simulink model "PIDRegulaceSS"  (R2020b)
settings: Solver=VariableStepAuto  StartTime=0.0  StopTime=inf  RelTol=1e-3
undefined symbols (not defined in the file): A_num, B_num, C, D, g, L
libraries: pid_lib x8, simulink x4
settings Model: Creator=kpass  LastModifiedBy=kpass

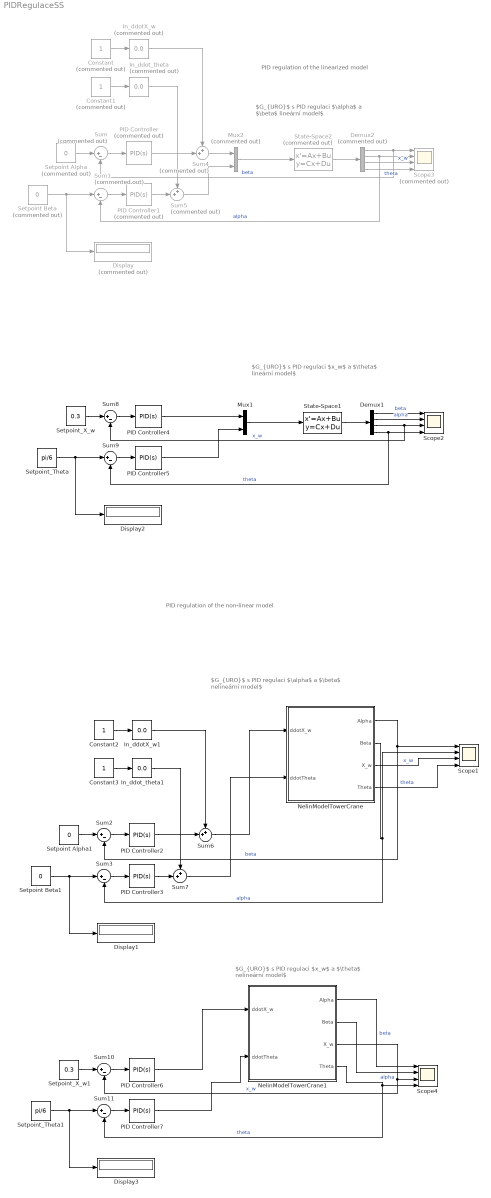
== system PIDRegulaceSS ==
  note: $G_{URO}$ s PID regulaci $x_w$ a $\theta$ nelineární model$
  note: PID regulation of the linearized model
  note: PID regulation of the non-linear model
  note: $G_{URO}$ s PID regulaci $x_w$ a $\theta$ lineární model$
  note: $G_{URO}$ s PID regulaci $\alpha$ a $\beta$ nelineární model$
  note: $G_{URO}$ s PID regulaci $\alpha$ a $\beta$ lineární model$
  Constant : Constant  Commented=on
  Constant1 : Constant  Commented=on
  Constant2 : Constant
  Constant3 : Constant
  Demux1 : Demux
  Demux2 : Demux  Commented=on
  Display : Display  Commented=on
  Display1 : Display
  Display2 : Display
  Display3 : Display
  In_ddotX_w : simulink/Math Operations/Slider Gain  Commented=on  gain=0.0  low=0  high=0.1
  In_ddotX_w1 : simulink/Math Operations/Slider Gain  gain=0.0  low=0  high=0.1
  In_ddot_theta : simulink/Math Operations/Slider Gain  Commented=on  gain=0.0  low=0  high=0.1
  In_ddot_theta1 : simulink/Math Operations/Slider Gain  gain=0.0  low=0  high=0.1
  Mux1 : Mux  Inputs=2
  Mux2 : Mux  Commented=on  Inputs=2
  NelinModelTowerCrane : Subsystem
  NelinModelTowerCrane1 : Subsystem
  PID Controller : pid_lib/PID Controller  Commented=on  Controller=PID  Form=Parallel  TimeDomain=Continuous-time  UseExternalTs=off  SampleTime=-1  IntegratorMethod=Forward Euler  FilterMethod=Forward Euler  ControllerParametersSource=internal  P=1  I=0  D=0  UseFilter=on  N=100  TunerSelectOption=Transfer Function Based (PID Tuner App)  InitialConditionSource=internal  InitialConditionForIntegrator=0  InitialConditionForFilter=0  DifferentiatorICPrevScaledInput=0  ExternalReset=none  TrackingMode=off  Kt=1  LimitOutput=off  SatLimitsSource=internal  UpperSaturationLimit=inf  LowerSaturationLimit=-inf  LinearizeAsGain=on  AntiWindupMode=none  Kb=1  POutMin=[]  POutMax=[]  IOutMin=[]  IOutMax=[]  DOutMin=[]  DOutMax=[]  NOutMin=[]  NOutMax=[]  SumOutMin=[]  SumOutMax=[]  SaturationOutMin=[]  SaturationOutMax=[]  PParamMin=[]  PParamMax=[]  IParamMin=[]  IParamMax=[]  DParamMin=[]  DParamMax=[]  NParamMin=[]  NParamMax=[]  KbParamMin=[]  KbParamMax=[]  KtParamMin=[]  KtParamMax=[]  KbOutMin=[]  KbOutMax=[]  KtOutMin=[]  KtOutMax=[]  IntegratorOutMin=[]  IntegratorOutMax=[]  FilterOutMin=[]  FilterOutMax=[]  SumI1OutMin=[]  SumI1OutMax=[]  SumI2OutMin=[]  SumI2OutMax=[]  SumI3OutMin=[]  SumI3OutMax=[]  SumI4OutMin=[]  SumI4OutMax=[]  SumDOutMin=[]  SumDOutMax=[]  DifferentiatorOutMin=[]  DifferentiatorOutMax=[]  FilterDiffOutCoefMin=[]  FilterDiffOutCoefMax=[]  ReciprocalOutMin=[]  ReciprocalOutMax=[]  SumDenOutMin=[]  SumDenOutMax=[]  SumNumOutMin=[]  SumNumOutMax=[]  DivideOutMin=[]  DivideOutMax=[]  UdiffTsProdOutMin=[]  UdiffTsProdOutMax=[]  NTsProdOutMin=[]  NTsProdOutMax=[]  UintegralTsProdOutMin=[]  UintegralTsProdOutMax=[]  UngainTsProdOutMin=[]  UngainTsProdOutMax=[]  IntegratorContinuousStateAttributes=''  IntegratorStateMustResolveToSignalObject=off  IntegratorRTWStateStorageClass=Auto  FilterContinuousStateAttributes=''  FilterStateMustResolveToSignalObject=off  FilterRTWStateStorageClass=Auto  ParallelPVariant=InternalParameters  IdealPVariant=Disabled  IVariant=InternalParameters  DVariant=InternalParameters  IntegratorVariant=Continuous  SatVariant=Disabled  AWVariant=Passthrough  PCopyVariant=Disabled  TRVariant=Disabled  FdbkBlocksVariant=Forward  IdealPFdbkVariant=Disabled  SatFdbkVariant=Disabled  DerivativeFilterVariant=ContFilter  NVariant=InternalParameters  NCopyVariant=Disabled  FilterICVariant=InternalICsFilter  IntegratorICVariant=InternalICs  ExternalResetVariant=Disabled  TRSumVariant=Passthrough  SumFdbkVariant=Disabled  SumVariant=Sum_PID  TsampFilterVariant=InternalTs  TsampNgainVariant=Passthrough  TsampIntegralVariant=Passthrough  ExternalSaturationOutDataTypeStr=Inherit: Same as second input
  PID Controller1 : pid_lib/PID Controller  Commented=on  Controller=PID  Form=Parallel  TimeDomain=Continuous-time  UseExternalTs=off  SampleTime=-1  IntegratorMethod=Forward Euler  FilterMethod=Forward Euler  ControllerParametersSource=internal  P=1  I=0  D=0  UseFilter=on  N=100  TunerSelectOption=Transfer Function Based (PID Tuner App)  InitialConditionSource=internal  InitialConditionForIntegrator=0  InitialConditionForFilter=0  DifferentiatorICPrevScaledInput=0  ExternalReset=none  TrackingMode=off  Kt=1  LimitOutput=off  SatLimitsSource=internal  UpperSaturationLimit=inf  LowerSaturationLimit=-inf  LinearizeAsGain=on  AntiWindupMode=none  Kb=1  POutMin=[]  POutMax=[]  IOutMin=[]  IOutMax=[]  DOutMin=[]  DOutMax=[]  NOutMin=[]  NOutMax=[]  SumOutMin=[]  SumOutMax=[]  SaturationOutMin=[]  SaturationOutMax=[]  PParamMin=[]  PParamMax=[]  IParamMin=[]  IParamMax=[]  DParamMin=[]  DParamMax=[]  NParamMin=[]  NParamMax=[]  KbParamMin=[]  KbParamMax=[]  KtParamMin=[]  KtParamMax=[]  KbOutMin=[]  KbOutMax=[]  KtOutMin=[]  KtOutMax=[]  IntegratorOutMin=[]  IntegratorOutMax=[]  FilterOutMin=[]  FilterOutMax=[]  SumI1OutMin=[]  SumI1OutMax=[]  SumI2OutMin=[]  SumI2OutMax=[]  SumI3OutMin=[]  SumI3OutMax=[]  SumI4OutMin=[]  SumI4OutMax=[]  SumDOutMin=[]  SumDOutMax=[]  DifferentiatorOutMin=[]  DifferentiatorOutMax=[]  FilterDiffOutCoefMin=[]  FilterDiffOutCoefMax=[]  ReciprocalOutMin=[]  ReciprocalOutMax=[]  SumDenOutMin=[]  SumDenOutMax=[]  SumNumOutMin=[]  SumNumOutMax=[]  DivideOutMin=[]  DivideOutMax=[]  UdiffTsProdOutMin=[]  UdiffTsProdOutMax=[]  NTsProdOutMin=[]  NTsProdOutMax=[]  UintegralTsProdOutMin=[]  UintegralTsProdOutMax=[]  UngainTsProdOutMin=[]  UngainTsProdOutMax=[]  IntegratorContinuousStateAttributes=''  IntegratorStateMustResolveToSignalObject=off  IntegratorRTWStateStorageClass=Auto  FilterContinuousStateAttributes=''  FilterStateMustResolveToSignalObject=off  FilterRTWStateStorageClass=Auto  ParallelPVariant=InternalParameters  IdealPVariant=Disabled  IVariant=InternalParameters  DVariant=InternalParameters  IntegratorVariant=Continuous  SatVariant=Disabled  AWVariant=Passthrough  PCopyVariant=Disabled  TRVariant=Disabled  FdbkBlocksVariant=Forward  IdealPFdbkVariant=Disabled  SatFdbkVariant=Disabled  DerivativeFilterVariant=ContFilter  NVariant=InternalParameters  NCopyVariant=Disabled  FilterICVariant=InternalICsFilter  IntegratorICVariant=InternalICs  ExternalResetVariant=Disabled  TRSumVariant=Passthrough  SumFdbkVariant=Disabled  SumVariant=Sum_PID  TsampFilterVariant=InternalTs  TsampNgainVariant=Passthrough  TsampIntegralVariant=Passthrough  ExternalSaturationOutDataTypeStr=Inherit: Same as second input
  PID Controller2 : pid_lib/PID Controller  Controller=PID  Form=Parallel  TimeDomain=Continuous-time  UseExternalTs=off  SampleTime=-1  IntegratorMethod=Forward Euler  FilterMethod=Forward Euler  ControllerParametersSource=internal  P=1  I=0  D=49.05  UseFilter=on  N=10  TunerSelectOption=Transfer Function Based (PID Tuner App)  InitialConditionSource=internal  InitialConditionForIntegrator=0  InitialConditionForFilter=0  DifferentiatorICPrevScaledInput=0  ExternalReset=none  TrackingMode=off  Kt=1  LimitOutput=off  SatLimitsSource=internal  UpperSaturationLimit=inf  LowerSaturationLimit=-inf  LinearizeAsGain=on  AntiWindupMode=none  Kb=1  POutMin=[]  POutMax=[]  IOutMin=[]  IOutMax=[]  DOutMin=[]  DOutMax=[]  NOutMin=[]  NOutMax=[]  SumOutMin=[]  SumOutMax=[]  SaturationOutMin=[]  SaturationOutMax=[]  PParamMin=[]  PParamMax=[]  IParamMin=[]  IParamMax=[]  DParamMin=[]  DParamMax=[]  NParamMin=[]  NParamMax=[]  KbParamMin=[]  KbParamMax=[]  KtParamMin=[]  KtParamMax=[]  KbOutMin=[]  KbOutMax=[]  KtOutMin=[]  KtOutMax=[]  IntegratorOutMin=[]  IntegratorOutMax=[]  FilterOutMin=[]  FilterOutMax=[]  SumI1OutMin=[]  SumI1OutMax=[]  SumI2OutMin=[]  SumI2OutMax=[]  SumI3OutMin=[]  SumI3OutMax=[]  SumI4OutMin=[]  SumI4OutMax=[]  SumDOutMin=[]  SumDOutMax=[]  DifferentiatorOutMin=[]  DifferentiatorOutMax=[]  FilterDiffOutCoefMin=[]  FilterDiffOutCoefMax=[]  ReciprocalOutMin=[]  ReciprocalOutMax=[]  SumDenOutMin=[]  SumDenOutMax=[]  SumNumOutMin=[]  SumNumOutMax=[]  DivideOutMin=[]  DivideOutMax=[]  UdiffTsProdOutMin=[]  UdiffTsProdOutMax=[]  NTsProdOutMin=[]  NTsProdOutMax=[]  UintegralTsProdOutMin=[]  UintegralTsProdOutMax=[]  UngainTsProdOutMin=[]  UngainTsProdOutMax=[]  IntegratorContinuousStateAttributes=''  IntegratorStateMustResolveToSignalObject=off  IntegratorRTWStateStorageClass=Auto  FilterContinuousStateAttributes=''  FilterStateMustResolveToSignalObject=off  FilterRTWStateStorageClass=Auto  ParallelPVariant=InternalParameters  IdealPVariant=Disabled  IVariant=InternalParameters  DVariant=InternalParameters  IntegratorVariant=Continuous  SatVariant=Disabled  AWVariant=Passthrough  PCopyVariant=Disabled  TRVariant=Disabled  FdbkBlocksVariant=Forward  IdealPFdbkVariant=Disabled  SatFdbkVariant=Disabled  DerivativeFilterVariant=ContFilter  NVariant=InternalParameters  NCopyVariant=Disabled  FilterICVariant=InternalICsFilter  IntegratorICVariant=InternalICs  ExternalResetVariant=Disabled  TRSumVariant=Passthrough  SumFdbkVariant=Disabled  SumVariant=Sum_PID  TsampFilterVariant=InternalTs  TsampNgainVariant=Passthrough  TsampIntegralVariant=Passthrough  ExternalSaturationOutDataTypeStr=Inherit: Same as second input
  PID Controller3 : pid_lib/PID Controller  Controller=PID  Form=Parallel  TimeDomain=Continuous-time  UseExternalTs=off  SampleTime=-1  IntegratorMethod=Forward Euler  FilterMethod=Forward Euler  ControllerParametersSource=internal  P=1  I=0  D=49.05  UseFilter=on  N=10  TunerSelectOption=Transfer Function Based (PID Tuner App)  InitialConditionSource=internal  InitialConditionForIntegrator=0  InitialConditionForFilter=0  DifferentiatorICPrevScaledInput=0  ExternalReset=none  TrackingMode=off  Kt=1  LimitOutput=off  SatLimitsSource=internal  UpperSaturationLimit=inf  LowerSaturationLimit=-inf  LinearizeAsGain=on  AntiWindupMode=none  Kb=1  POutMin=[]  POutMax=[]  IOutMin=[]  IOutMax=[]  DOutMin=[]  DOutMax=[]  NOutMin=[]  NOutMax=[]  SumOutMin=[]  SumOutMax=[]  SaturationOutMin=[]  SaturationOutMax=[]  PParamMin=[]  PParamMax=[]  IParamMin=[]  IParamMax=[]  DParamMin=[]  DParamMax=[]  NParamMin=[]  NParamMax=[]  KbParamMin=[]  KbParamMax=[]  KtParamMin=[]  KtParamMax=[]  KbOutMin=[]  KbOutMax=[]  KtOutMin=[]  KtOutMax=[]  IntegratorOutMin=[]  IntegratorOutMax=[]  FilterOutMin=[]  FilterOutMax=[]  SumI1OutMin=[]  SumI1OutMax=[]  SumI2OutMin=[]  SumI2OutMax=[]  SumI3OutMin=[]  SumI3OutMax=[]  SumI4OutMin=[]  SumI4OutMax=[]  SumDOutMin=[]  SumDOutMax=[]  DifferentiatorOutMin=[]  DifferentiatorOutMax=[]  FilterDiffOutCoefMin=[]  FilterDiffOutCoefMax=[]  ReciprocalOutMin=[]  ReciprocalOutMax=[]  SumDenOutMin=[]  SumDenOutMax=[]  SumNumOutMin=[]  SumNumOutMax=[]  DivideOutMin=[]  DivideOutMax=[]  UdiffTsProdOutMin=[]  UdiffTsProdOutMax=[]  NTsProdOutMin=[]  NTsProdOutMax=[]  UintegralTsProdOutMin=[]  UintegralTsProdOutMax=[]  UngainTsProdOutMin=[]  UngainTsProdOutMax=[]  IntegratorContinuousStateAttributes=''  IntegratorStateMustResolveToSignalObject=off  IntegratorRTWStateStorageClass=Auto  FilterContinuousStateAttributes=''  FilterStateMustResolveToSignalObject=off  FilterRTWStateStorageClass=Auto  ParallelPVariant=InternalParameters  IdealPVariant=Disabled  IVariant=InternalParameters  DVariant=InternalParameters  IntegratorVariant=Continuous  SatVariant=Disabled  AWVariant=Passthrough  PCopyVariant=Disabled  TRVariant=Disabled  FdbkBlocksVariant=Forward  IdealPFdbkVariant=Disabled  SatFdbkVariant=Disabled  DerivativeFilterVariant=ContFilter  NVariant=InternalParameters  NCopyVariant=Disabled  FilterICVariant=InternalICsFilter  IntegratorICVariant=InternalICs  ExternalResetVariant=Disabled  TRSumVariant=Passthrough  SumFdbkVariant=Disabled  SumVariant=Sum_PID  TsampFilterVariant=InternalTs  TsampNgainVariant=Passthrough  TsampIntegralVariant=Passthrough  ExternalSaturationOutDataTypeStr=Inherit: Same as second input
  PID Controller{4..7} (4 alike) : pid_lib/PID Controller  Controller=PID  Form=Parallel  TimeDomain=Continuous-time  UseExternalTs=off  SampleTime=-1  IntegratorMethod=Forward Euler  FilterMethod=Forward Euler  ControllerParametersSource=internal  P=1  I=0  D=2  UseFilter=on  N=100  TunerSelectOption=Transfer Function Based (PID Tuner App)  InitialConditionSource=internal  InitialConditionForIntegrator=0  InitialConditionForFilter=0  DifferentiatorICPrevScaledInput=0  ExternalReset=none  TrackingMode=off  Kt=1  LimitOutput=off  SatLimitsSource=internal  UpperSaturationLimit=inf  LowerSaturationLimit=-inf  LinearizeAsGain=on  AntiWindupMode=none  Kb=1  POutMin=[]  POutMax=[]  IOutMin=[]  IOutMax=[]  DOutMin=[]  DOutMax=[]  NOutMin=[]  NOutMax=[]  SumOutMin=[]  SumOutMax=[]  SaturationOutMin=[]  SaturationOutMax=[]  PParamMin=[]  PParamMax=[]  IParamMin=[]  IParamMax=[]  DParamMin=[]  DParamMax=[]  NParamMin=[]  NParamMax=[]  KbParamMin=[]  KbParamMax=[]  KtParamMin=[]  KtParamMax=[]  KbOutMin=[]  KbOutMax=[]  KtOutMin=[]  KtOutMax=[]  IntegratorOutMin=[]  IntegratorOutMax=[]  FilterOutMin=[]  FilterOutMax=[]  SumI1OutMin=[]  SumI1OutMax=[]  SumI2OutMin=[]  SumI2OutMax=[]  SumI3OutMin=[]  SumI3OutMax=[]  SumI4OutMin=[]  SumI4OutMax=[]  SumDOutMin=[]  SumDOutMax=[]  DifferentiatorOutMin=[]  DifferentiatorOutMax=[]  FilterDiffOutCoefMin=[]  FilterDiffOutCoefMax=[]  ReciprocalOutMin=[]  ReciprocalOutMax=[]  SumDenOutMin=[]  SumDenOutMax=[]  SumNumOutMin=[]  SumNumOutMax=[]  DivideOutMin=[]  DivideOutMax=[]  UdiffTsProdOutMin=[]  UdiffTsProdOutMax=[]  NTsProdOutMin=[]  NTsProdOutMax=[]  UintegralTsProdOutMin=[]  UintegralTsProdOutMax=[]  UngainTsProdOutMin=[]  UngainTsProdOutMax=[]  IntegratorContinuousStateAttributes=''  IntegratorStateMustResolveToSignalObject=off  IntegratorRTWStateStorageClass=Auto  FilterContinuousStateAttributes=''  FilterStateMustResolveToSignalObject=off  FilterRTWStateStorageClass=Auto  ParallelPVariant=InternalParameters  IdealPVariant=Disabled  IVariant=InternalParameters  DVariant=InternalParameters  IntegratorVariant=Continuous  SatVariant=Disabled  AWVariant=Passthrough  PCopyVariant=Disabled  TRVariant=Disabled  FdbkBlocksVariant=Forward  IdealPFdbkVariant=Disabled  SatFdbkVariant=Disabled  DerivativeFilterVariant=ContFilter  NVariant=InternalParameters  NCopyVariant=Disabled  FilterICVariant=InternalICsFilter  IntegratorICVariant=InternalICs  ExternalResetVariant=Disabled  TRSumVariant=Passthrough  SumFdbkVariant=Disabled  SumVariant=Sum_PID  TsampFilterVariant=InternalTs  TsampNgainVariant=Passthrough  TsampIntegralVariant=Passthrough  ExternalSaturationOutDataTypeStr=Inherit: Same as second input
  Scope1 : Scope  NumInputPorts=4
  Scope2 : Scope  NumInputPorts=4
  Scope3 : Scope  Commented=on  NumInputPorts=4
  Scope4 : Scope  NumInputPorts=4
  Setpoint Alpha : Constant  Commented=on  Value=0
  Setpoint Alpha1 : Constant  Value=0
  Setpoint Beta : Constant  Commented=on  Value=0
  Setpoint Beta1 : Constant  Value=0
  Setpoint_Theta : Constant  Value=pi/6
  Setpoint_Theta1 : Constant  Value=pi/6
  Setpoint_X_w : Constant  Value=0.3
  Setpoint_X_w1 : Constant  Value=0.3
  State-Space1 : StateSpace  A=A_num  B=B_num  C=C  D=D  InitialCondition=[0 0 0 0 0 0 0 0]
  State-Space2 : StateSpace  Commented=on  A=A_num  B=B_num  C=C  D=D  InitialCondition=[0 0 0 0 0 0 0 0]
  Sum : Sum  Commented=on  Inputs=|+-
  Sum1 : Sum  Commented=on  Inputs=|+-
  Sum{2..3,8..11} (6 alike) : Sum  Inputs=|+-
  Sum4 : Sum  Commented=on  Inputs=++|
  Sum5 : Sum  Commented=on  Inputs=++|
  Sum6 : Sum  Inputs=++|
  Sum7 : Sum  Inputs=++|
  wires:
  Mux2/1 -> State-Space2/1
  Demux2/2 -> Scope3/2, Sum1/2  "alpha"
  State-Space2/1 -> Demux2/1
  Demux2/3 -> Scope3/3  "x_w"
  Setpoint Alpha/1 -> Sum/1
  Sum1/1 -> PID Controller1/1
  Demux2/4 -> Scope3/4  "theta"
  Demux2/1 -> Sum/2, Scope3/1  "beta"
  Sum/1 -> PID Controller/1
  Setpoint Beta/1 -> Display/1, Sum1/1
  Constant/1 -> In_ddotX_w/1
  PID Controller/1 -> Sum4/2
  Sum4/1 -> Mux2/1
  In_ddotX_w/1 -> Sum4/1
  PID Controller1/1 -> Sum5/2
  Sum5/1 -> Mux2/2
  Constant1/1 -> In_ddot_theta/1
  In_ddot_theta/1 -> Sum5/1
  Sum7/1 -> NelinModelTowerCrane/2(ddotTheta)
  In_ddot_theta1/1 -> Sum7/1
  PID Controller3/1 -> Sum7/2
  Constant2/1 -> In_ddotX_w1/1
  Sum6/1 -> NelinModelTowerCrane/1(ddotX_w)
  In_ddotX_w1/1 -> Sum6/1
  NelinModelTowerCrane/4(Theta) -> Scope1/4  "theta"
  PID Controller2/1 -> Sum6/2
  NelinModelTowerCrane/3(X_w) -> Scope1/3  "x_w"
  NelinModelTowerCrane/2(Beta) -> Scope1/2, Sum3/2  "alpha"
  NelinModelTowerCrane/1(Alpha) -> Sum2/2, Scope1/1  "beta"
  Setpoint Beta1/1 -> Display1/1, Sum3/1
  Sum2/1 -> PID Controller2/1
  Sum3/1 -> PID Controller3/1
  Constant3/1 -> In_ddot_theta1/1
  Setpoint Alpha1/1 -> Sum2/1
  PID Controller5/1 -> Mux1/2
  PID Controller4/1 -> Mux1/1
  Demux1/4 -> Scope2/4, Sum9/2  "theta"
  Demux1/3 -> Scope2/3, Sum8/2  "x_w"
  Demux1/2 -> Scope2/2  "alpha"
  Demux1/1 -> Scope2/1  "beta"
  Setpoint_Theta/1 -> Display2/1, Sum9/1
  Sum8/1 -> PID Controller4/1
  Sum9/1 -> PID Controller5/1
  State-Space1/1 -> Demux1/1
  Setpoint_X_w/1 -> Sum8/1
  Mux1/1 -> State-Space1/1
  PID Controller7/1 -> NelinModelTowerCrane1/2(ddotTheta)
  PID Controller6/1 -> NelinModelTowerCrane1/1(ddotX_w)
  Setpoint_X_w1/1 -> Sum10/1
  Setpoint_Theta1/1 -> Display3/1, Sum11/1
  Sum10/1 -> PID Controller6/1
  Sum11/1 -> PID Controller7/1
  NelinModelTowerCrane1/1(Alpha) -> Scope4/1  "beta"
  NelinModelTowerCrane1/2(Beta) -> Scope4/2  "alpha"
  NelinModelTowerCrane1/4(Theta) -> Scope4/4, Sum11/2  "theta"
  NelinModelTowerCrane1/3(X_w) -> Scope4/3, Sum10/2  "x_w"

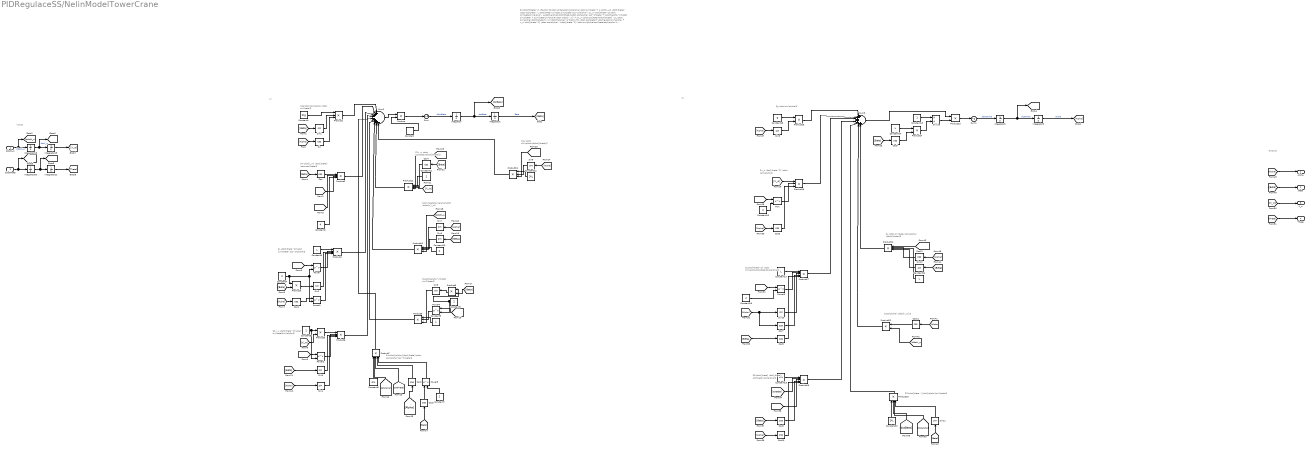
== system PIDRegulaceSS/NelinModelTowerCrane ==
  note: 2)
  note: $L \cdot sin(\beta) cos(\alpha) \ddot{\theta}$
  note: $cos(\alpha) \ddot{x_w}$
  note: $2L\dot{\beta}\dot{\alpha}sin(\beta)$
  note: $2L\dot{\beta} \dot{\theta} cos(\beta) cos(\alpha)$
  note: $L\dot{\theta^2} \cdot sin(\alpha)cos(\beta)cos(\alpha)$
  note: $x_w \dot{\theta^2} \cdot cos(\alpha)$
  note: $g \cdot sin(\alpha)$
  note: Inputs
  note: 1)
  note: $2L \cdot sin(\alpha)\ddot{\theta}$
  note: $2x_w \cdot cos(\beta)\ddot{\theta}$
  note: $2sin(\beta)sin(\alpha)\cdot \ddot{x}_w$
  note: $L\dot{\alpha^2}\cdot sin(2\beta)$
  note: $4L\dot{\alpha}\dot{\theta}\cdot cos(\alpha) cos^2(\beta)$
  note: $2x_w \dot{\theta^2}\cdot sin(\beta)sin(\alpha)$
  note: $L \dot{\theta^2}\cdot sin(2\beta) cos^2(\alpha)$
  note: $4 \dot{x_w} \dot{\theta} \cdot cos(\beta)$
  note: $2g\cdot cos(\alpha) \cdot sin(\beta)$
  note: $1)\ddot{\beta} = -\frac{1}{2\cdot L}(2g\cdot cos(\alpha) \cdot sin(\beta) + 4 \dot{x_w} \dot{\theta} \cdot cos(\beta) - L \dot{\theta^2}\cdot sin(2\beta) cos^2(\alpha) - 2x_w \dot{\theta^2}\cdot sin(\beta)sin(\alpha) - 4L\dot{\alpha}\dot{\theta}\cdot cos(\alpha) cos^2(\beta) + L\dot{\alpha^2}\cdot sin(2\beta) + 2sin(\beta)sin(\alpha)\cdot \ddot{x_w} + 2x_w \cdot cos(\beta)\ddot{\theta} - 2L \cdot sin(\alpha)\ddot{\theta}) \\ 2) \ddot{\alpha} = \frac{1}{L \cdot cos(\beta)} \cdot (g\cdot sin(\alpha) + x_w \dot{\theta^2} \cdot cos(\alpha) - L\dot{\theta^2} \cdot sin(\alpha)cos(\beta)cos(\alpha) + 2L\dot{\beta} \dot{\theta} cos(\beta) cos(\alpha) - 2L\dot{\beta}\dot{\alpha}sin(\beta) - cos(\alpha) \ddot{x_w} + L \cdot sin(\beta) cos(\alpha) \ddot{\theta})$
  note: Outputs
  ddotX_w : Inport
  ddotTheta : Inport  Port=2
  Constant : Constant  Value=1/(2*L)
  Constant1 : Constant  Value=2*g
  Constant{4..5,7,9..11,16,18} (8 alike) : Constant  Value=2
  Constant12 : Constant  Value=2*L
  Constant13 : Constant
  Constant{3,8,14,17,21} (5 alike) : Constant  Value=L
  Constant15 : Constant  Value=g
  Constant19 : Constant  Value=2*L
  Constant2 : Constant  Value=4
  Constant20 : Constant  Value=2*L
  Constant6 : Constant  Value=4*L
  Cos{,1..12} (13 alike) : Trigonometry  Operator=cos
  Divide : Product  Inputs=*/
  Integrator{,1..3,18,20..21} (7 alike) : Integrator
  Integrator19 : Integrator  InitialCondition=0.1  LimitOutput=on  UpperSaturationLimit=0.6  LowerSaturationLimit=0
  Pow : Math  Operator=pow  RndMeth=Zero  SaturateOnIntegerOverflow=on
  Power{,1..5} (6 alike) : Math  Operator=pow  SaturateOnIntegerOverflow=on
  Product{,3,5,8,13..15,20} (8 alike) : Product
  Product{1,9,12,16} (4 alike) : Product  Inputs=3
  Product{2,4,6,10..11,19,21} (7 alike) : Product  Inputs=4
  Product17 : Product  Inputs=5
  Product18 : Product  Inputs=5
  Product7 : Product  Inputs=5
  Sin : Trigonometry  Operator=cos
  Sin{1..12} (12 alike) : Trigonometry
  Sum : Sum  Inputs=-
  Sum1 : Sum  Inputs=-
  Sum2 : Sum  Inputs=|++---+++-
  Sum3 : Sum  Inputs=|++-+--+
  Alpha : Outport
  Beta : Outport  Port=2
  X_w : Outport  Port=3
  Theta : Outport  Port=4
  wires:
  Sin/1 -> Product1/3
  Constant1/1 -> Product1/1
  Integrator1/1 -> [Beta]  "Beta"
  Sin1/1 -> Product1/2
  Integrator3/1 -> [Alpha]  "Alpha"
  Sum/1 -> Integrator/1  "ddotBeta"
  Integrator2/1 -> [dotAlpha], Integrator3/1  "dotAlpha"
  Product1/1 -> Sum2/1
  Integrator/1 -> [dotBeta], Integrator1/1  "dotBeta"
  Sum1/1 -> Integrator2/1  "ddotAlpha"
  Constant/1 -> Product/2
  Sum2/1 -> Product/1
  Product/1 -> Sum/1
  [Beta] -> Sin1/1
  [Alpha] -> Sin/1
  [Beta] -> Cos/1
  Cos/1 -> Product2/1
  [dotX_w] -> Product2/3
  [dotTheta] -> Product2/2
  Constant2/1 -> Product2/4
  Product2/1 -> Sum2/2
  [dotTheta] -> Power/1
  Constant4/1 -> Power1/2, Power/2, Product3/1
  [Beta] -> Product3/2
  Product3/1 -> Sin2/1
  [Alpha] -> Cos1/1
  Cos1/1 -> Power1/1
  Constant3/1 -> Product4/1
  Power/1 -> Product4/2
  Sin2/1 -> Product4/3
  Power1/1 -> Product4/4
  Product4/1 -> Sum2/3
  Constant5/1 -> Product5/1, Power2/2
  [X_w] -> Product5/2
  [dotTheta] -> Power2/1
  [Beta] -> Sin3/1
  [Alpha] -> Sin4/1
  Product5/1 -> Product6/1
  Power2/1 -> Product6/2
  Sin3/1 -> Product6/3
  Sin4/1 -> Product6/4
  Product6/1 -> Sum2/4
  Constant7/1 -> Power3/2
  Cos3/1 -> Power3/1
  [Beta] -> Cos3/1
  [Alpha] -> Cos2/1
  Constant6/1 -> Product7/1
  [dotAlpha] -> Product7/2
  [dotTheta] -> Product7/3
  Cos2/1 -> Product7/4
  Power3/1 -> Product7/5
  Product7/1 -> Sum2/5
  [dotAlpha] -> Power4/1
  Constant9/1 -> Product8/1, Power4/2
  [Beta] -> Product8/2
  Product8/1 -> Sin5/1
  Constant8/1 -> Product9/1
  Power4/1 -> Product9/2
  Sin5/1 -> Product9/3
  Product9/1 -> Sum2/6
  Constant10/1 -> Product10/1
  Sin6/1 -> Product10/2
  Sin7/1 -> Product10/3
  [ddotX_w] -> Product10/4
  [Beta] -> Sin6/1
  [Alpha] -> Sin7/1
  Product10/1 -> Sum2/7
  [Beta] -> Cos4/1
  [X_w] -> Product11/1
  Constant11/1 -> Product11/2
  Cos4/1 -> Product11/3
  [ddotTheta] -> Product11/4
  Product11/1 -> Sum2/8
  [Alpha] -> Sin8/1
  Constant12/1 -> Product12/1
  Sin8/1 -> Product12/2
  [ddotTheta] -> Product12/3
  Product12/1 -> Sum2/9
  Product13/1 -> Sum1/1
  Divide/1 -> Product13/2
  Constant13/1 -> Divide/1
  Product14/1 -> Divide/2
  Constant14/1 -> Product14/1
  Cos5/1 -> Product14/2
  [Beta] -> Cos5/1
  Sum3/1 -> Product13/1
  [Alpha] -> Sin9/1
  Constant15/1 -> Product15/1
  Sin9/1 -> Product15/2
  Product15/1 -> Sum3/1
  [dotTheta] -> Pow/1
  Constant16/1 -> Pow/2
  [Alpha] -> Cos6/1
  [X_w] -> Product16/1
  Pow/1 -> Product16/2
  Cos6/1 -> Product16/3
  Product16/1 -> Sum3/2
  [dotTheta] -> Power5/1
  Constant18/1 -> Power5/2
  [Alpha] -> Cos7/1, Sin10/1
  [Beta] -> Cos8/1
  Constant17/1 -> Product17/1
  Power5/1 -> Product17/2
  Sin10/1 -> Product17/3
  Cos7/1 -> Product17/4
  Cos8/1 -> Product17/5
  Product17/1 -> Sum3/3
  [Beta] -> Cos9/1
  [Alpha] -> Cos10/1
  Constant19/1 -> Product18/1
  [dotBeta] -> Product18/2
  [dotTheta] -> Product18/3
  Cos9/1 -> Product18/4
  Cos10/1 -> Product18/5
  Product18/1 -> Sum3/4
  [Beta] -> Sin11/1
  Constant20/1 -> Product19/1
  [dotBeta] -> Product19/2
  [dotAlpha] -> Product19/3
  Sin11/1 -> Product19/4
  Product19/1 -> Sum3/5
  [Alpha] -> Cos11/1
  Cos11/1 -> Product20/1
  [ddotX_w] -> Product20/2
  Product20/1 -> Sum3/6
  [Beta] -> Sin12/1
  [Alpha] -> Cos12/1
  [ddotTheta] -> Product21/1
  Cos12/1 -> Product21/2
  Sin12/1 -> Product21/4
  Constant21/1 -> Product21/3
  Product21/1 -> Sum3/7
  ddotX_w/1 -> Integrator18/1, [ddotX_w]  "ddotX_w"
  Integrator18/1 -> [dotX_w], Integrator19/1  "dotX_w"
  Integrator19/1 -> [X_w]
  ddotTheta/1 -> [ddotTheta], Integrator20/1
  Integrator20/1 -> [dotTheta], Integrator21/1
  Integrator21/1 -> [Theta]
  [Beta] -> Beta/1
  [Theta] -> Theta/1
  [Alpha] -> Alpha/1
  [X_w] -> X_w/1

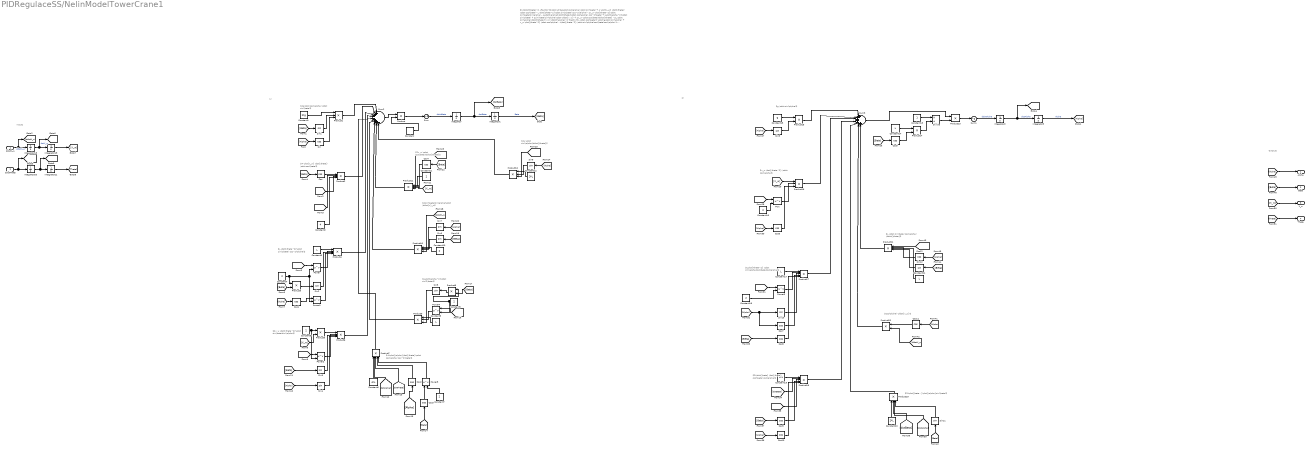
== system PIDRegulaceSS/NelinModelTowerCrane1 ==
  note: 2)
  note: $L \cdot sin(\beta) cos(\alpha) \ddot{\theta}$
  note: $cos(\alpha) \ddot{x_w}$
  note: $2L\dot{\beta}\dot{\alpha}sin(\beta)$
  note: $2L\dot{\beta} \dot{\theta} cos(\beta) cos(\alpha)$
  note: $L\dot{\theta^2} \cdot sin(\alpha)cos(\beta)cos(\alpha)$
  note: $x_w \dot{\theta^2} \cdot cos(\alpha)$
  note: $g \cdot sin(\alpha)$
  note: Inputs
  note: 1)
  note: $2L \cdot sin(\alpha)\ddot{\theta}$
  note: $2x_w \cdot cos(\beta)\ddot{\theta}$
  note: $2sin(\beta)sin(\alpha)\cdot \ddot{x}_w$
  note: $L\dot{\alpha^2}\cdot sin(2\beta)$
  note: $4L\dot{\alpha}\dot{\theta}\cdot cos(\alpha) cos^2(\beta)$
  note: $2x_w \dot{\theta^2}\cdot sin(\beta)sin(\alpha)$
  note: $L \dot{\theta^2}\cdot sin(2\beta) cos^2(\alpha)$
  note: $4 \dot{x_w} \dot{\theta} \cdot cos(\beta)$
  note: $2g\cdot cos(\alpha) \cdot sin(\beta)$
  note: $1)\ddot{\beta} = -\frac{1}{2\cdot L}(2g\cdot cos(\alpha) \cdot sin(\beta) + 4 \dot{x_w} \dot{\theta} \cdot cos(\beta) - L \dot{\theta^2}\cdot sin(2\beta) cos^2(\alpha) - 2x_w \dot{\theta^2}\cdot sin(\beta)sin(\alpha) - 4L\dot{\alpha}\dot{\theta}\cdot cos(\alpha) cos^2(\beta) + L\dot{\alpha^2}\cdot sin(2\beta) + 2sin(\beta)sin(\alpha)\cdot \ddot{x_w} + 2x_w \cdot cos(\beta)\ddot{\theta} - 2L \cdot sin(\alpha)\ddot{\theta}) \\ 2) \ddot{\alpha} = \frac{1}{L \cdot cos(\beta)} \cdot (g\cdot sin(\alpha) + x_w \dot{\theta^2} \cdot cos(\alpha) - L\dot{\theta^2} \cdot sin(\alpha)cos(\beta)cos(\alpha) + 2L\dot{\beta} \dot{\theta} cos(\beta) cos(\alpha) - 2L\dot{\beta}\dot{\alpha}sin(\beta) - cos(\alpha) \ddot{x_w} + L \cdot sin(\beta) cos(\alpha) \ddot{\theta})$
  note: Outputs
  ddotX_w : Inport
  ddotTheta : Inport  Port=2
  Constant : Constant  Value=1/(2*L)
  Constant1 : Constant  Value=2*g
  Constant{4..5,7,9..11,16,18} (8 alike) : Constant  Value=2
  Constant12 : Constant  Value=2*L
  Constant13 : Constant
  Constant{3,8,14,17,21} (5 alike) : Constant  Value=L
  Constant15 : Constant  Value=g
  Constant19 : Constant  Value=2*L
  Constant2 : Constant  Value=4
  Constant20 : Constant  Value=2*L
  Constant6 : Constant  Value=4*L
  Cos{,1..12} (13 alike) : Trigonometry  Operator=cos
  Divide : Product  Inputs=*/
  Integrator{,1..3,18,20..21} (7 alike) : Integrator
  Integrator19 : Integrator  InitialCondition=0.1  LimitOutput=on  UpperSaturationLimit=0.6  LowerSaturationLimit=0
  Pow : Math  Operator=pow  RndMeth=Zero  SaturateOnIntegerOverflow=on
  Power{,1..5} (6 alike) : Math  Operator=pow  SaturateOnIntegerOverflow=on
  Product{,3,5,8,13..15,20} (8 alike) : Product
  Product{1,9,12,16} (4 alike) : Product  Inputs=3
  Product{2,4,6,10..11,19,21} (7 alike) : Product  Inputs=4
  Product17 : Product  Inputs=5
  Product18 : Product  Inputs=5
  Product7 : Product  Inputs=5
  Sin : Trigonometry  Operator=cos
  Sin{1..12} (12 alike) : Trigonometry
  Sum : Sum  Inputs=-
  Sum1 : Sum  Inputs=-
  Sum2 : Sum  Inputs=|++---+++-
  Sum3 : Sum  Inputs=|++-+--+
  Alpha : Outport
  Beta : Outport  Port=2
  X_w : Outport  Port=3
  Theta : Outport  Port=4
  wires:
  Sin/1 -> Product1/3
  Constant1/1 -> Product1/1
  Integrator1/1 -> [Beta]  "Beta"
  Sin1/1 -> Product1/2
  Integrator3/1 -> [Alpha]  "Alpha"
  Sum/1 -> Integrator/1  "ddotBeta"
  Integrator2/1 -> [dotAlpha], Integrator3/1  "dotAlpha"
  Product1/1 -> Sum2/1
  Integrator/1 -> [dotBeta], Integrator1/1  "dotBeta"
  Sum1/1 -> Integrator2/1  "ddotAlpha"
  Constant/1 -> Product/2
  Sum2/1 -> Product/1
  Product/1 -> Sum/1
  [Beta] -> Sin1/1
  [Alpha] -> Sin/1
  [Beta] -> Cos/1
  Cos/1 -> Product2/1
  [dotX_w] -> Product2/3
  [dotTheta] -> Product2/2
  Constant2/1 -> Product2/4
  Product2/1 -> Sum2/2
  [dotTheta] -> Power/1
  Constant4/1 -> Power1/2, Power/2, Product3/1
  [Beta] -> Product3/2
  Product3/1 -> Sin2/1
  [Alpha] -> Cos1/1
  Cos1/1 -> Power1/1
  Constant3/1 -> Product4/1
  Power/1 -> Product4/2
  Sin2/1 -> Product4/3
  Power1/1 -> Product4/4
  Product4/1 -> Sum2/3
  Constant5/1 -> Product5/1, Power2/2
  [X_w] -> Product5/2
  [dotTheta] -> Power2/1
  [Beta] -> Sin3/1
  [Alpha] -> Sin4/1
  Product5/1 -> Product6/1
  Power2/1 -> Product6/2
  Sin3/1 -> Product6/3
  Sin4/1 -> Product6/4
  Product6/1 -> Sum2/4
  Constant7/1 -> Power3/2
  Cos3/1 -> Power3/1
  [Beta] -> Cos3/1
  [Alpha] -> Cos2/1
  Constant6/1 -> Product7/1
  [dotAlpha] -> Product7/2
  [dotTheta] -> Product7/3
  Cos2/1 -> Product7/4
  Power3/1 -> Product7/5
  Product7/1 -> Sum2/5
  [dotAlpha] -> Power4/1
  Constant9/1 -> Product8/1, Power4/2
  [Beta] -> Product8/2
  Product8/1 -> Sin5/1
  Constant8/1 -> Product9/1
  Power4/1 -> Product9/2
  Sin5/1 -> Product9/3
  Product9/1 -> Sum2/6
  Constant10/1 -> Product10/1
  Sin6/1 -> Product10/2
  Sin7/1 -> Product10/3
  [ddotX_w] -> Product10/4
  [Beta] -> Sin6/1
  [Alpha] -> Sin7/1
  Product10/1 -> Sum2/7
  [Beta] -> Cos4/1
  [X_w] -> Product11/1
  Constant11/1 -> Product11/2
  Cos4/1 -> Product11/3
  [ddotTheta] -> Product11/4
  Product11/1 -> Sum2/8
  [Alpha] -> Sin8/1
  Constant12/1 -> Product12/1
  Sin8/1 -> Product12/2
  [ddotTheta] -> Product12/3
  Product12/1 -> Sum2/9
  Product13/1 -> Sum1/1
  Divide/1 -> Product13/2
  Constant13/1 -> Divide/1
  Product14/1 -> Divide/2
  Constant14/1 -> Product14/1
  Cos5/1 -> Product14/2
  [Beta] -> Cos5/1
  Sum3/1 -> Product13/1
  [Alpha] -> Sin9/1
  Constant15/1 -> Product15/1
  Sin9/1 -> Product15/2
  Product15/1 -> Sum3/1
  [dotTheta] -> Pow/1
  Constant16/1 -> Pow/2
  [Alpha] -> Cos6/1
  [X_w] -> Product16/1
  Pow/1 -> Product16/2
  Cos6/1 -> Product16/3
  Product16/1 -> Sum3/2
  [dotTheta] -> Power5/1
  Constant18/1 -> Power5/2
  [Alpha] -> Cos7/1, Sin10/1
  [Beta] -> Cos8/1
  Constant17/1 -> Product17/1
  Power5/1 -> Product17/2
  Sin10/1 -> Product17/3
  Cos7/1 -> Product17/4
  Cos8/1 -> Product17/5
  Product17/1 -> Sum3/3
  [Beta] -> Cos9/1
  [Alpha] -> Cos10/1
  Constant19/1 -> Product18/1
  [dotBeta] -> Product18/2
  [dotTheta] -> Product18/3
  Cos9/1 -> Product18/4
  Cos10/1 -> Product18/5
  Product18/1 -> Sum3/4
  [Beta] -> Sin11/1
  Constant20/1 -> Product19/1
  [dotBeta] -> Product19/2
  [dotAlpha] -> Product19/3
  Sin11/1 -> Product19/4
  Product19/1 -> Sum3/5
  [Alpha] -> Cos11/1
  Cos11/1 -> Product20/1
  [ddotX_w] -> Product20/2
  Product20/1 -> Sum3/6
  [Beta] -> Sin12/1
  [Alpha] -> Cos12/1
  [ddotTheta] -> Product21/1
  Cos12/1 -> Product21/2
  Sin12/1 -> Product21/4
  Constant21/1 -> Product21/3
  Product21/1 -> Sum3/7
  ddotX_w/1 -> Integrator18/1, [ddotX_w]  "ddotX_w"
  Integrator18/1 -> [dotX_w], Integrator19/1  "dotX_w"
  Integrator19/1 -> [X_w]
  ddotTheta/1 -> [ddotTheta], Integrator20/1
  Integrator20/1 -> [dotTheta], Integrator21/1
  Integrator21/1 -> [Theta]
  [Beta] -> Beta/1
  [Theta] -> Theta/1
  [Alpha] -> Alpha/1
  [X_w] -> X_w/1
